simulink model "HIL_Testing_SW_amantest"  (Simulink 7.5)
settings: Solver=ode1  StartTime=0.0  StopTime=Inf  FixedStep=0.001  RelTol=1e-3
PostLoadFcn:
  | , if any(exist('dsrtsu_mdlpostloadfcn', 'file') == [2, 3, 6]), try dsrtsu_mdlpostloadfcn('Execute', bdroot); catch fprintf('Error in PostLoadFcn (dsrtsu_mdlpostloadfcn) for model "%s":\n %s\n', bdroot, lasterr); end, end,
undefined symbols (not defined in the file): CeBSER_Cnt_NumTempAxisPts, ChargeCord, ChargeCord_Control, ChargeToSOCCurr, ChrgCurrLim, CrntSens1Fine, CS_SOCSetPt, CyclerMaxChrgPwr, CyclerMaxDschrgPwr, deltaAhr, Drive_1, Drive_10, Drive_11, Drive_12, Drive_13, Drive_14, Drive_15, Drive_16, Drive_17, Drive_18, Drive_19, Drive_2, Drive_20, Drive_21, Drive_22, Drive_23, Drive_24, Drive_25, Drive_26, Drive_27, Drive_28, Drive_29, Drive_3, Drive_30, Drive_31, Drive_32, Drive_33, Drive_34, Drive_35, Drive_36, Drive_37, Drive_38, Drive_39, Drive_4, Drive_40, Drive_41, Drive_42, Drive_43, Drive_44, Drive_45, Drive_46, Drive_47, Drive_48, Drive_49, Drive_5, Drive_50, Drive_51, Drive_6, Drive_7, Drive_8 ... (+50)
libraries: simulink x129, rtican x50, rti2211sailib x5, rti2211serlib x5, rti2202miolib x3
(part 12 of 23)

== system HIL_Testing_SW_amantest/TX/Tx_Cycler/Send Remote Request B ==
  note: 0x01C3
  Control : Inport  OutDataType=sfix(16)  OutScaling=2^0
  StationID_B1 : Inport  Port=2  OutDataType=sfix(16)  OutScaling=2^0
  StationID_B : Inport  Port=3  OutDataType=sfix(16)  OutScaling=2^0
  Hardware_Version : Inport  Port=4  OutDataType=sfix(16)  OutScaling=2^0
  Enable : EnablePort
  Bus Selector7 : BusSelector  OutputSignals=Channel_Change_B,Control_From_B,Control_To_B
  Change_Control_B : rtican/RTICAN Transmit (TX)   SystemSampleTime=-1  Reserved1=[]  Reserved2=[]  Reserved3=[]  Reserved4=[]  SfcnMessage=[]  Msg_Struct=[]  BoardTypeNo=[]  BoardNo=[]  ChannelNo=[]  Parameters=[]  DialogFcn=[]  UnitName=[]  Revision=[]  UnitValues=[]  DSProperties=struct('RTI',struct('Version',uint32(5),'BlockType',struct('isSLSource',uint8(1),'isSLSink',uint8(1),'isHWSource',uint8(0),'isHWSink',uint8(0),'isSetup',uint8(0),'isInline',uint8(1),'isNonInline',uint8(0),'isInterrupt',uint8(0),'isChannelwise',uint8(0)),'IOBoardType','RTICAN','UnitType','MESSAGE','Identifier','TX','DialogType','MSVC','BlockSet','RTICAN','SlaveProcessor','CAN'))  RTIBlockInterface=struct('InputPortsWidth',int32([1 1 1 1 1 1]),'InputPortsActive',[1 1 1 1 1 1],'InputPortsName',{{'CC_channel_change_B','CC_control_from_B','CC_control_to_B','Station_ID_B','Hardware_ver_ID_B','Station_IDA_B'}},'InputPortsDataType',{{'SS_DOUBLE','SS_DOUBLE','SS_DOUBLE','SS_DOUBLE','SS_DOUBLE','SS_DOUBLE'}},'OutputPortsWidth',int32(1),'OutputPortsActive',1,'OutputPortsName',{{['TX status']}},'DialogFcn','rtican_message_interface_gui','BlockDisplay',{{'','center'}},'IconTransparency','on','InitLevel',3,'BlockName',struct('Token',{{'Change_Control_B'}}),'SampleTime',{{-1}},'TriggerPort',{{'none'}},'EnablePort',{{'none'}})  RTIBlockParameters=struct('BoardTypeNo',{{2211,'OFF',[]}},'BoardNo',{{2,'ON',[1 16]}},'ChannelNo',{{1,'ON',[1 2]}},'Parameters',{{struct('DataFileSupport',struct('DataFileSelectedMaster',1,'DataFileSelectedLocal',1,'DataFileName','c:\data\testing\av900_dbc\av900_mod.dbc|','DataFileDate',{{{['20-Apr-2011 08:23:37']}}},'SelectedFile','av900_dbc\av900_mod.dbc','InterfaceFcn','rtican_dbc_file_parser'),'Options',struct('StatusSelected',1,'TimeSelected',0,'DeltaTimeSelected',0,'DelayTimeSelected',0,'DelayTimeTXCommandSelected',0,'EncodeSetUnusedBitsToOne',0,'EnableMsgLoopback',0,'TriggerPort',struct('Selected',0,'TriggerType',0),'EnablePortSelected',0,'SignalOnPortnameSelected',1,'UserCoding',struct('Selected',0,'InterfaceFile','UserEncodingFile','FcnName','UserEncodeFcn','InportSelected',0,'InportWidth',1,'OutportSelected',0,'OutportWidth',1),'TerminationMsg',struct('Selected',0,'Byte0_7','0'),'InitialMsg',struct('Selected',0,'Byte0_7','0')),'Message',struct('MsgOnBlocknameSelected',1,'MsgName','Change_Control_B','MsgIdFormat',0,'MsgId',451,'MsgLength',8,'NumSignals',6,'SampleTime',-1,'StartTime',struct('Selected',0,'Value',0),'AutoRepeatTime',struct('Selected',0,'Value',0.1),'Timeout',struct('Selected',0,'Value',0.1),'DelayTime',struct('Selected',0,'Value',0.1),'Signal',struct('SgnName',{'CC_channel_change_B','CC_control_from_B','CC_control_to_B','Station_ID_B','Hardware_ver_ID_B','Station_IDA_B'},'SgnStartBit',{0,1,4,8,8,56},'SgnLength',{1,3,3,32,16,8},'SgnType',{0,0,0,0,0,0},'ModeValue',{-1,-1,-1,-1,-1,-1},'DataType',{0,0,0,0,0,0},'ByteLayout',{0,0,0,2,0,0},'Factor',{1,1,1,1,1,1},'Offset',{0,0,0,0,0,0},'SgnComment',{{''},{''},{''},{''},{''},{''}},'SgnUnit',{'code','code','code','code','code','code'},'Min',{0,0,0,0,0,0},'Max',{1,7,7,0,65535,255},'SLDataType',{'SS_DOUBLE','SS_DOUBLE','SS_DOUBLE','SS_DOUBLE','SS_DOUBLE','SS_DOUBLE'}),'MsgIdNumFormat',0,'MsgComment',{{''}}),'Version',1.2,'general',struct('isFromLib',0)),'OFF',[]}},'GroupId',{{struct('Group',{{'RTICAN'}},'No',6,'Behavior',{{'NAMECHANGE'}},'BlockType',{{'SINK'}},'NameChangeFlag',0),'OFF',[]}},'SFcnRTICANMessage',{{struct('MsgType','TX','SFcnPortType','Scalar','MsgName','Change_Control_B','MsgIdFormat','STD','MsgId',451,'MsgLength',8,'NumSignals',6,'SampleTime',-1,'StartTime',struct('Selected','no','Value',0),'AutoRepeatTime',struct('Selected','no','Value',0.1),'Timeout',struct('Selected','no','Value',0.1),'Signal',struct('SgnName',{'CC_channel_change_B','CC_control_from_B','CC_control_to_B','Station_ID_B','Hardware_ver_ID_B','Station_IDA_B'},'SgnStartBit',{0,1,4,8,8,56},'SgnLength',{1,3,3,32,16,8},'SgnType',{'standard','standard','standard','standard','standard','standard'},'ModeValue',{-1,-1,-1,-1,-1,-1},'DataType',{['unsigned int'],['unsigned int'],['unsigned int'],['unsigned int'],['unsigned int'],['unsigned int']},'ByteLayout',{['little endian'],['little endian'],['little endian'],['motorola back.'],['little endian'],['little endian']},'Factor',{1,1,1,1,1,1},'Offset',{0,0,0,0,0,0},'SLDataType',{'SS_DOUBLE','SS_DOUBLE','SS_DOUBLE','SS_DOUBLE','SS_DOUBLE','SS_DOUBLE'}),'StatusSelected','yes','TimeSelected','no','DeltaTimeSelected','no','DelayTimeSelected','no','DelayTimeTXCommandSelected','no','EncodeSetUnusedBitsToOne','no','EnableMsgLoopback','no','TriggerPort',struct('Selected','no','TriggerType',0),'EnablePortSelected','no','UserCoding',struct('Selected','no','InterfaceFile','UserEncodingFile','FcnName','UserEncodeFcn','InportSelected','no','InportWidth',1,'OutportSelected','no','OutportWidth',1),'TerminationMsg',struct('Selected','no','Byte0','0x00','Byte1','0x00','Byte2','0x00','Byte3','0x00','Byte4','0x00','Byte5','0x00','Byte6','0x00','Byte7','0x00'),'InitialMsg',struct('Selected','no','Byte0','0x00','Byte1','0x00','Byte2','0x00','Byte3','0x00','Byte4','0x00','Byte5','0x00','Byte6','0x00','Byte7','0x00'),'BoardType','DS2211','BoardNo',2,'ControllerNo',1),'OFF',[]}},'TLCFileName',{{'rtican_tx_message','OFF',[]}})  RTISFcnParameters=struct('SFcnRTICANMessage','struct','TLCFileName','char')  RTIBlockParaDefault=struct('BoardTypeNo',4302,'BoardNo',1,'ChannelNo',1,'Parameters',struct('DataFileSupport',struct('DataFileSelectedMaster',0,'DataFileSelectedLocal',0,'DataFileName','','DataFileDate','','SelectedFile',['<no file selected>']),'Options',struct('StatusSelected',1,'TimeSelected',1,'DeltaTimeSelected',1,'DelayTimeSelected',1,'DelayTimeTXCommandSelected',0,'EncodeSetUnusedBitsToOne',0,'EnableMsgLoopback',0,'TriggerPort',struct('Selected',0,'TriggerType','rising'),'EnablePortSelected',0,'SignalOnPortnameSelected',1,'UserCoding',struct('Selected',0,'InterfaceFile','UserEncodingFile','FcnName','UserEncodeFcn','InportSelected',0,'InportWidth',1,'OutportSelected',0,'OutportWidth',1),'TerminationMsg',struct('Selected',0,'Byte0_7','0'),'InitialMsg',struct('Selected',0,'Byte0_7','0')),'Message',struct('MsgOnBlocknameSelected',0,'MsgName',['TX Message'],'MsgIdFormat',0,'MsgId',100,'MsgLength',8,'NumSignals',1,'SampleTime',-1,'StartTime',struct('Selected',0,'Value',0),'AutoRepeatTime',struct('Selected',0,'Value',0.1),'Timeout',struct('Selected',0,'Value',0.1),'DelayTime',struct('Selected',0,'Value',0.1),'Signal',struct('SgnName',['TX signal'],'SgnStartBit',0,'SgnLength',8,'SgnType',0,'ModeValue',-1,'DataType',0,'SLDataType','SS_DOUBLE','ByteLayout',0,'Factor',1,'Offset',0,'Min',0,'Max',255,'SgnComment',{{}},'SgnUnit',''),'MsgIdNumFormat',0,'MsgComment',{{''}}),'Version',1.2,'general',struct('isFromLib',1)),'GroupId',struct('Group',{{'RTICAN'}},'No',1,'Behavior',{{'NAMECHANGE'}},'BlockType',{{'SINK'}},'NameChangeFlag',0),'SFcnRTICANMessage',struct('MsgType','TX','MsgName',['TX Message'],'MsgIdFormat','STD','MsgId',100,'MsgLength',2,'NumSignals',1,'SampleTime',-1,'StartTime',struct('Selected','no','Value',0),'AutoRepeatTime',struct('Selected','no','Value',0.1),'Timeout',struct('Selected','no','Value',0.1),'DelayTime',struct('Selected','no','Value',0.1),'Signal',struct('SgnName',['TX signal'],'SgnStartBit',0,'SgnLength',8,'SgnType','standard','ModeValue',-1,'DataType',['unsigned int'],'ByteLayout',['little endian'],'SLDataType','SS_DOUBLE','Factor',1,'Offset',0),'StatusSelected','yes','TimeSelected','yes','DeltaTimeSelected','yes','DelayTimeSelected','yes','EnablePortSelected','no','EnableMsgLoopback','no','DelayTimeTXCommandSelected','no','EncodeSetUnusedBitsToOne','no','UserCoding',struct('Selected','no','InterfaceFile','UserDecodingFile','FcnName','UserDecodeFcn','InportSelected','no','InportWidth',1,'OutportSelected','no','OutportWidth',1),'TerminationMsg',struct('Selected','no','Byte0','0x00','Byte1','0x00','Byte2','0x00','Byte3','0x00','Byte4','0x00','Byte5','0x00','Byte6','0x00','Byte7','0x00'),'InitialMsg',struct('Selected','no','Byte0','0x00','Byte1','0x00','Byte2','0x00','Byte3','0x00','Byte4','0x00','Byte5','0x00','Byte6','0x00','Byte7','0x00'),'TriggerPort',struct('Selected','no','TriggerType','rising'),'BoardType','DS4302','BoardNo',1,'ControllerNo',1,'SFcnPortType','Scalar'),'TLCFileName','rtican_tx_message')
      settings: AttributesFormatString=Group Id: RTICAN6\n
  Constant : Constant  OutDataType=sfix(16)  OutScaling=2^0
  Data Store Write1 : DataStoreWrite  DataStoreName=Remote_Req_B_Sent  SampleTime=-1
  Data Type Conversion{1..5,7} (6 alike) : DataTypeConversion  OutDataType=fixdt(1, 16)  OutScaling=2^0
  Terminator : Terminator
  wires:
  Bus Selector7/1 -> Data Type Conversion7/1  "<Channel_Change_B>"
  Bus Selector7/2 -> Data Type Conversion1/1  "<Control_From_B>"
  Bus Selector7/3 -> Data Type Conversion2/1  "<Control_To_B>"
  StationID_B1/1 -> Data Type Conversion5/1
  Hardware_Version/1 -> Data Type Conversion4/1
  StationID_B/1 -> Data Type Conversion3/1
  Change_Control_B/1 -> Terminator/1
  Control/1 -> Bus Selector7/1
  Constant/1 -> Data Store Write1/1
  Data Type Conversion7/1 -> Change_Control_B/1
  Data Type Conversion1/1 -> Change_Control_B/2
  Data Type Conversion2/1 -> Change_Control_B/3
  Data Type Conversion3/1 -> Change_Control_B/4
  Data Type Conversion4/1 -> Change_Control_B/5
  Data Type Conversion5/1 -> Change_Control_B/6

== system HIL_Testing_SW_amantest/TX/Tx_Cycler/Subsystem ==
  In : Inport
  0x140_Latch_Reset : Constant  Value=0  OutDataType=sfix(16)  OutScaling=2^0
  Comparison4 : RelationalOperator  Operator===  LogicOutDataTypeMode=boolean  OutDataTypeStr=boolean
  Constant Value : Constant  Value=single(1)  OutDataType=sfix(16)  OutScaling=2^0
  Data Type Conversion : DataTypeConversion  OutDataType=sfix(16)  OutScaling=2^0
  Data Type Conversion1 : DataTypeConversion  OutDataType=sfix(16)  OutScaling=2^0
  OurLatchReset : Subsystem
  Out : Outport
  wires:
  OurLatchReset/1(Out1) -> Data Type Conversion/1
  Constant Value/1 -> Comparison4/2
  Comparison4/1 -> OurLatchReset/1(U)
  In/1 -> Comparison4/1
  Data Type Conversion/1 -> Out/1
  Data Type Conversion1/1 -> OurLatchReset/2(Reset)
  0x140_Latch_Reset/1 -> Data Type Conversion1/1

== system HIL_Testing_SW_amantest/TX/Tx_Cycler/TX_ABC_ChA ==
  Control_Value : Inport  OutDataType=sfix(16)  OutScaling=2^0
  Control_Mode : Inport  Port=2  OutDataType=sfix(16)  OutScaling=2^0
  Enable : EnablePort
  Chart : Stateflow chart  TreatAsAtomicUnit=on
  TickTick : Constant  Value=10  OutDataType=sfix(16)  OutScaling=2^0
  msg_0x1A0_Command_A : Subsystem  TreatAsAtomicUnit=on
  msg_0x1A1_Low_Lim_A_out : Subsystem  TreatAsAtomicUnit=on
  msg_0x1A2_Upp_Lim_A_out : Subsystem  TreatAsAtomicUnit=on
  wires:
  Control_Mode/1 -> msg_0x1A0_Command_A/3(Control_Mode)
  Control_Value/1 -> msg_0x1A0_Command_A/2(Control_Value_Proc)
  Chart/3(Trigger_three) -> msg_0x1A2_Upp_Lim_A_out/Enable
  Chart/2(Trigger_two) -> msg_0x1A1_Low_Lim_A_out/Enable
  Chart/1(Trigger_one) -> msg_0x1A0_Command_A/Enable
  Chart/4(Increment) -> [Counter]
  [Counter] -> msg_0x1A2_Upp_Lim_A_out/1(Counter)
  [Counter] -> msg_0x1A1_Low_Lim_A_out/1(Counter)
  [Counter] -> msg_0x1A0_Command_A/1(Counter)
  TickTick/1 -> Chart/1(TickTick)

== system HIL_Testing_SW_amantest/TX/Tx_Cycler/TX_ABC_ChB ==
  Control_Value : Inport  OutDataType=sfix(16)  OutScaling=2^0
  Control_Mode : Inport  Port=2  OutDataType=sfix(16)  OutScaling=2^0
  Enable : EnablePort
  Chart : Stateflow chart  TreatAsAtomicUnit=on
  TickTick : Constant  Value=10  OutDataType=sfix(16)  OutScaling=2^0
  msg_0x1A0_Command_B : Subsystem  TreatAsAtomicUnit=on
  msg_0x1A1_Low_Lim_B_out : Subsystem  TreatAsAtomicUnit=on
  msg_0x1A2_Upp_Lim_B_out : Subsystem  TreatAsAtomicUnit=on
  wires:
  TickTick/1 -> Chart/1(TickTick)
  [Counter] -> msg_0x1A0_Command_B/1(Counter)
  [Counter] -> msg_0x1A1_Low_Lim_B_out/1(Counter)
  [Counter] -> msg_0x1A2_Upp_Lim_B_out/1(Counter)
  Chart/4(Increment) -> [Counter]
  Chart/1(Trigger_one) -> msg_0x1A0_Command_B/Enable
  Chart/2(Trigger_two) -> msg_0x1A1_Low_Lim_B_out/Enable
  Chart/3(Trigger_three) -> msg_0x1A2_Upp_Lim_B_out/Enable
  Control_Value/1 -> msg_0x1A0_Command_B/2(Control_Value_Proc)
  Control_Mode/1 -> msg_0x1A0_Command_B/3(Control_Mode)

== system HIL_Testing_SW_amantest/HWO/TX HVEM/ChargeCord_Control/110 ==
  Action Port : ActionPort  ActionType=then
  Constant : Constant  OutDataTypeMode=uint32  OutDataType=sfix(16)  OutScaling=2^0  OutDataTypeStr=uint32
  Out1 : Outport  OutDataType=sfix(16)  OutScaling=2^0  InitialOutput=1
  wires:
  Constant/1 -> Out1/1

== system HIL_Testing_SW_amantest/HWO/TX HVEM/ChargeCord_Control/220 ==
  Action Port : ActionPort  ActionType=elseif
  Constant : Constant  Value=2  OutDataTypeMode=uint32  OutDataType=sfix(16)  OutScaling=2^0  OutDataTypeStr=uint32
  Out1 : Outport  OutDataType=sfix(16)  OutScaling=2^0  InitialOutput=2
  wires:
  Constant/1 -> Out1/1

== system HIL_Testing_SW_amantest/HWO/TX HVEM/ChargeCord_Control/Cord Connected ==
  Proximity : Inport  OutDataType=sfix(16)  OutScaling=2^0
  Freq1 : Inport  Port=2  OutDataType=sfix(16)  OutScaling=2^0
  AC_Enable : Inport  Port=3  OutDataType=sfix(16)  OutScaling=2^0
  Outlet Type : Inport  Port=4  OutDataType=sfix(16)  OutScaling=2^0
  PrcsdVolt_Freq1 : Inport  Port=5  OutDataType=sfix(16)  OutScaling=2^0
  Action Port : ActionPort  ActionType=then
  110 Connected : Subsystem  TreatAsAtomicUnit=on
  110_Current : Constant  Value=11  OutDataType=sfix(16)  OutScaling=2^0  OutDataTypeStr=Inherit: Inherit via back propagation
  110_DC : Constant  Value=20  OutDataType=sfix(16)  OutScaling=2^0  OutDataTypeStr=Inherit: Inherit via back propagation
  110_Temp : Constant  Value=22  OutDataType=sfix(16)  OutScaling=2^0  OutDataTypeStr=Inherit: Inherit via back propagation
  110_Volts : Constant  Value=110  OutDataType=sfix(16)  OutScaling=2^0  OutDataTypeStr=Inherit: Inherit via back propagation
  220 Connected : Subsystem  TreatAsAtomicUnit=on
  220_Current : Constant  Value=15  OutDataType=sfix(16)  OutScaling=2^0  OutDataTypeStr=Inherit: Inherit via back propagation
  220_DC : Constant  Value=22  OutDataType=sfix(16)  OutScaling=2^0  OutDataTypeStr=Inherit: Inherit via back propagation
  220_Temp : Constant  Value=22  OutDataType=sfix(16)  OutScaling=2^0  OutDataTypeStr=Inherit: Inherit via back propagation
  220_Volts : Constant  Value=220  OutDataType=sfix(16)  OutScaling=2^0  OutDataTypeStr=Inherit: Inherit via back propagation
  AC Enabled : Subsystem  TreatAsAtomicUnit=on
  AC Not Enabled : Subsystem  TreatAsAtomicUnit=on
  ACNotEnableD_Current : Constant  Value=0  OutDataType=sfix(16)  OutScaling=2^0  OutDataTypeStr=Inherit: Inherit via back propagation
  ACNotEnabled_Volts : Constant  Value=0  OutDataType=sfix(16)  OutScaling=2^0  OutDataTypeStr=Inherit: Inherit via back propagation
  If1 : If  IfExpression=u1==1  ElseIfExpressions=u1==2  ZeroCross=off
  If2 : If  IfExpression=u1==1  ZeroCross=off
  Merge{,1..3,6} (5 alike) : Merge  Inputs=3
  Merge4 : Merge
  Merge5 : Merge
  Not Connected : Subsystem  TreatAsAtomicUnit=on
  NotConnecteD_Temp : Constant  Value=-40  OutDataType=sfix(16)  OutScaling=2^0  OutDataTypeStr=Inherit: Inherit via back propagation
  NotConnected_Current : Constant  Value=0  OutDataType=sfix(16)  OutScaling=2^0  OutDataTypeStr=Inherit: Inherit via back propagation
  NotConnected_DC : Constant  Value=10  OutDataType=sfix(16)  OutScaling=2^0  OutDataTypeStr=Inherit: Inherit via back propagation
  NotConnected_Volts : Constant  Value=0  OutDataType=sfix(16)  OutScaling=2^0  OutDataTypeStr=Inherit: Inherit via back propagation
  ChargeCrdPresent : Outport  OutDataType=sfix(16)  OutScaling=2^0
  DC : Outport  Port=2  OutDataType=sfix(16)  OutScaling=2^0
  Freq : Outport  Port=3  OutDataType=sfix(16)  OutScaling=2^0
  Voltage : Outport  Port=4  OutDataType=sfix(16)  OutScaling=2^0  InitialOutput=0
  Current : Outport  Port=5  OutDataType=sfix(16)  OutScaling=2^0  InitialOutput=0
  Temp : Outport  Port=6  OutDataType=sfix(16)  OutScaling=2^0
  PrcsdVolt_DC : Outport  Port=7  OutDataType=sfix(16)  OutScaling=2^0
  PrcsdVolt_Freq : Outport  Port=8  OutDataType=sfix(16)  OutScaling=2^0
  wires:
  If2/1 -> AC Enabled/Action
  AC Not Enabled/2(Current_out) -> Merge5/2
  AC Not Enabled/1(Volt_out) -> Merge4/2
  ACNotEnableD_Current/1 -> AC Not Enabled/2(Current_in)
  ACNotEnabled_Volts/1 -> AC Not Enabled/1(Volt_in)
  If1/1 -> 110 Connected/Action
  [Current] -> AC Enabled/2(Current_in)
  [Voltage] -> AC Enabled/1(Volt_in)
  Merge1/1 -> [Current]
  Merge/1 -> [Voltage]
  AC Enabled/2(Current_out) -> Merge5/1
  AC Enabled/1(Volt_out) -> Merge4/1
  Merge5/1 -> Current/1
  Merge4/1 -> Voltage/1
  Merge3/1 -> DC/1
  Merge2/1 -> Temp/1
  If2/2 -> AC Not Enabled/Action
  AC_Enable/1 -> If2/1
  Proximity/1 -> ChargeCrdPresent/1
  Freq1/1 -> Freq/1
  Outlet Type/1 -> If1/1
  110_Volts/1 -> 110 Connected/1(Volt_in)
  If1/2 -> 220 Connected/Action
  If1/3 -> Not Connected/Action
  110_Current/1 -> 110 Connected/2(Current_in)
  110_Temp/1 -> 110 Connected/3(Temp_in)
  220_Volts/1 -> 220 Connected/1(Volt_in)
  220_Current/1 -> 220 Connected/2(Current_in)
  220_Temp/1 -> 220 Connected/3(Temp_in)
  NotConnected_Volts/1 -> Not Connected/1(Volt_in)
  NotConnected_Current/1 -> Not Connected/2(Current_in)
  NotConnecteD_Temp/1 -> Not Connected/3(Temp_in)
  110 Connected/1(Volt_out) -> Merge/1
  110 Connected/2(Current_out) -> Merge1/1
  220 Connected/1(Volt_out) -> Merge/2
  220 Connected/2(Current_out) -> Merge1/2
  110 Connected/3(Temp_out) -> Merge2/1
  220 Connected/3(Temp_out) -> Merge2/2
  Not Connected/1(Volt_out) -> Merge/3
  Not Connected/2(Current_out) -> Merge1/3
  Not Connected/3(Temp_out) -> Merge2/3
  220_DC/1 -> 220 Connected/4(DC_in)
  110 Connected/4(DC_Out) -> Merge3/1
  110_DC/1 -> 110 Connected/4(DC_in)
  220 Connected/4(DC_Out) -> Merge3/2
  NotConnected_DC/1 -> Not Connected/4(DC_in)
  Not Connected/4(DC_Out) -> Merge3/3
  Merge6/1 -> PrcsdVolt_DC/1
  110 Connected/5(PrcsdVolt_DC) -> Merge6/1
  220 Connected/5(PrcsdVolt_DC) -> Merge6/2
  Not Connected/5(PrcsdVolt_DC) -> Merge6/3
  PrcsdVolt_Freq1/1 -> PrcsdVolt_Freq/1

== system HIL_Testing_SW_amantest/HWO/TX HVEM/ChargeCord_Control/Cord Not Connected ==
  Proximity : Inport  OutDataType=sfix(16)  OutScaling=2^0
  DC_in : Inport  Port=2  OutDataType=sfix(16)  OutScaling=2^0
  Freq_in : Inport  Port=3  OutDataType=sfix(16)  OutScaling=2^0
  Voltage_in : Inport  Port=4  OutDataType=sfix(16)  OutScaling=2^0
  Current_in : Inport  Port=5  OutDataType=sfix(16)  OutScaling=2^0
  Temp_in : Inport  Port=6  OutDataType=sfix(16)  OutScaling=2^0
  PrcsdVolt_DC_in : Inport  Port=7  OutDataType=sfix(16)  OutScaling=2^0
  PrcsdVolt_Freq_in : Inport  Port=8  OutDataType=sfix(16)  OutScaling=2^0
  Action Port : ActionPort  ActionType=else
  ChargeCrdPresent : Outport  OutDataType=sfix(16)  OutScaling=2^0
  DC_out : Outport  Port=2  OutDataType=sfix(16)  OutScaling=2^0
  Freq : Outport  Port=3  OutDataType=sfix(16)  OutScaling=2^0
  Voltage : Outport  Port=4  OutDataType=sfix(16)  OutScaling=2^0
  Current : Outport  Port=5  OutDataType=sfix(16)  OutScaling=2^0
  Temp : Outport  Port=6  OutDataType=sfix(16)  OutScaling=2^0
  PrcsdVolt_DC : Outport  Port=7  OutDataType=sfix(16)  OutScaling=2^0
  PrcsdVolt_Freq : Outport  Port=8  OutDataType=sfix(16)  OutScaling=2^0
  wires:
  Temp_in/1 -> Temp/1
  Current_in/1 -> Current/1
  Freq_in/1 -> Freq/1
  Voltage_in/1 -> Voltage/1
  Proximity/1 -> ChargeCrdPresent/1
  DC_in/1 -> DC_out/1
  PrcsdVolt_DC_in/1 -> PrcsdVolt_DC/1
  PrcsdVolt_Freq_in/1 -> PrcsdVolt_Freq/1

== system HIL_Testing_SW_amantest/HWO/TX HVEM/ChargeCord_Control/Disconnected ==
  Action Port : ActionPort  ActionType=else
  Constant : Constant  Value=0  OutDataTypeMode=uint32  OutDataType=sfix(16)  OutScaling=2^0  OutDataTypeStr=uint32
  Out1 : Outport  OutDataType=sfix(16)  OutScaling=2^0  InitialOutput=3
  wires:
  Constant/1 -> Out1/1

== system HIL_Testing_SW_amantest/HWO/TX HVEM/ChargeCord_Control/OurLatchReset ==
  U : Inport  OutDataType=fixdt(1, 16)  OutScaling=2^0
  Reset : Inport  Port=2  OutDataType=fixdt(1, 16)  OutScaling=2^0
  Logical Operator : Logic  Operator=NOT  AllPortsSameDT=off  OutDataTypeMode=boolean  LogicDataType=fixdt(0, 8)  OutDataTypeStr=boolean
  Logical Operator1 : Logic  Operator=OR  AllPortsSameDT=off  OutDataTypeMode=boolean  LogicDataType=fixdt(0, 8)  OutDataTypeStr=boolean
  Logical Operator2 : Logic  AllPortsSameDT=off  OutDataTypeMode=boolean  LogicDataType=fixdt(0, 8)  OutDataTypeStr=boolean
  Unit Delay : UnitDelay  SampleTime=-1
  Out1 : Outport  OutDataType=fixdt(1, 16)  OutScaling=2^0
  wires:
  Unit Delay/1 -> Logical Operator2/2
  Logical Operator1/1 -> Unit Delay/1, Out1/1
  U/1 -> Logical Operator1/1
  Logical Operator2/1 -> Logical Operator1/2
  Logical Operator/1 -> Logical Operator2/1
  Reset/1 -> Logical Operator/1

== system HIL_Testing_SW_amantest/HWO/TX HVEM/ChargeCord_Control/OurLatchReset1 ==
  U : Inport  OutDataType=fixdt(1, 16)  OutScaling=2^0
  Reset : Inport  Port=2  OutDataType=fixdt(1, 16)  OutScaling=2^0
  Logical Operator : Logic  Operator=NOT  AllPortsSameDT=off  OutDataTypeMode=boolean  LogicDataType=fixdt(0, 8)  OutDataTypeStr=boolean
  Logical Operator1 : Logic  Operator=OR  AllPortsSameDT=off  OutDataTypeMode=boolean  LogicDataType=fixdt(0, 8)  OutDataTypeStr=boolean
  Logical Operator2 : Logic  AllPortsSameDT=off  OutDataTypeMode=boolean  LogicDataType=fixdt(0, 8)  OutDataTypeStr=boolean
  Unit Delay : UnitDelay  SampleTime=-1
  Out1 : Outport  OutDataType=fixdt(1, 16)  OutScaling=2^0
  wires:
  Reset/1 -> Logical Operator/1
  Logical Operator/1 -> Logical Operator2/1
  Logical Operator2/1 -> Logical Operator1/2
  U/1 -> Logical Operator1/1
  Logical Operator1/1 -> Out1/1, Unit Delay/1
  Unit Delay/1 -> Logical Operator2/2

== system HIL_Testing_SW_amantest/LionsHeart/FeaturePresentation/Ahr_Integration/Clear Ahr ==
  note: Clear Ahr
  Enable : EnablePort
  Constant Value{,1..3} (4 alike) : Constant  Value=0  OutDataType=sfix(16)  OutScaling=2^0
  Data Store Write : DataStoreWrite  DataStoreName=Ahr  SampleTime=-1
  Data Store Write1 : DataStoreWrite  DataStoreName=Whr  SampleTime=-1
  Data Store Write2 : DataStoreWrite  DataStoreName=Whr_PackSens  SampleTime=-1
  Data Store Write3 : DataStoreWrite  DataStoreName=Ahr_PackSens  SampleTime=-1
  wires:
  Constant Value/1 -> Data Store Write/1
  Constant Value1/1 -> Data Store Write1/1
  Constant Value2/1 -> Data Store Write2/1
  Constant Value3/1 -> Data Store Write3/1

== system HIL_Testing_SW_amantest/LionsHeart/FeaturePresentation/Ahr_Integration/Cycler_Ahr ==
  Current : Inport  OutDataType=sfix(16)  OutScaling=2^0
  Voltage : Inport  Port=2  OutDataType=sfix(16)  OutScaling=2^0
  Constant Value : Constant  Value=0.001  OutDataType=sfix(16)  OutScaling=2^0
  Constant Value1 : Constant  Value=3600  OutDataType=sfix(16)  OutScaling=2^0
  Data Store Read1 : DataStoreRead  DataStoreName=SOC  SampleTime=0
  Data Store Read2 : DataStoreRead  DataStoreName=PackCapacity  SampleTime=0
  Data Store Read3 : DataStoreRead  DataStoreName=Ahr  SampleTime=0
  Data Store Read4 : DataStoreRead  DataStoreName=Whr  SampleTime=0
  Divide : Constant  Value=2  OutDataType=sfix(16)  OutScaling=2^0
  Product : Product  OutDataType=sfix(16)  OutScaling=2^0  RndMeth=Zero
  Product1 : Product  Inputs=*/  OutDataType=sfix(16)  OutScaling=2^0  RndMeth=Zero
  Product2 : Product  Inputs=*/  OutDataType=sfix(16)  OutScaling=2^0  RndMeth=Zero
  Product3 : Product  Inputs=*/  OutDataType=sfix(16)  OutScaling=2^0  RndMeth=Zero
  Product4 : Product  OutDataType=sfix(16)  OutScaling=2^0  RndMeth=Zero
  Sum{,1..3} (4 alike) : Sum  OutDataType=sfix(16)  OutScaling=2^0  RndMeth=Zero
  Unit Delay : UnitDelay  SampleTime=-1
  SOC : Outport  OutDataType=fixdt(1, 16)  OutScaling=2^0
  Ahr : Outport  Port=2  OutDataType=fixdt(1, 16)  OutScaling=2^0
  Whr : Outport  Port=3  OutDataType=fixdt(1, 16)  OutScaling=2^0
  wires:
  [Inst_SOC] -> Sum2/1
  Product2/1 -> Product/1
  Constant Value/1 -> Product/2
  Product/1 -> Product1/1
  Constant Value1/1 -> Product1/2
  Divide/1 -> Product2/2
  Sum1/1 -> Product2/1
  Current/1 -> Sum1/1, Unit Delay/1
  Unit Delay/1 -> Sum1/2
  Product1/1 -> Sum/1, Product3/1, Product4/1
  Product3/1 -> [Inst_SOC]
  Data Store Read2/1 -> Product3/2
  Sum/1 -> Ahr/1
  Voltage/1 -> Product4/2
  Product4/1 -> Sum3/1
  Sum3/1 -> Whr/1
  Data Store Read1/1 -> Sum2/2
  Sum2/1 -> SOC/1
  Data Store Read3/1 -> Sum/2
  Data Store Read4/1 -> Sum3/2

== system HIL_Testing_SW_amantest/LionsHeart/FeaturePresentation/Ahr_Integration/Lookup_SOC ==
  note: SOC Reset
  Voltage : Inport  OutDataType=sfix(16)  OutScaling=2^0
  BatTemp : Inport  Port=2  OutDataType=sfix(16)  OutScaling=2^0
  PackVoltage : Inport  Port=3  OutDataType=sfix(16)  OutScaling=2^0
  Enable : EnablePort
  Data Store Read1 : DataStoreRead  DataStoreName=NumberOfCells  SampleTime=-1
  Data Store Read2 : DataStoreRead  DataStoreName=NumberOfCells  SampleTime=-1
  Data Store Write1 : DataStoreWrite  DataStoreName=SOC  SampleTime=-1
  Data Store Write2 : DataStoreWrite  DataStoreName=SOC_PackSens  SampleTime=-1
  Data Type Conversion{1..2,5..6} (4 alike) : DataTypeConversion  OutDataTypeMode=single  OutDataType=sfix(16)  OutScaling=2^0  OutDataTypeStr=single
  Data Type Conversion3 : DataTypeConversion  OutDataTypeMode=double  OutDataType=sfix(16)  OutScaling=2^0  OutDataTypeStr=double
  Data Type Conversion4 : DataTypeConversion  OutDataTypeMode=double  OutDataType=sfix(16)  OutScaling=2^0  OutDataTypeStr=double
  Divide1 : Product  Inputs=*/  OutDataType=sfix(16)  OutScaling=2^-10
  Divide2 : Product  Inputs=*/  OutDataType=sfix(16)  OutScaling=2^-10
  OCV_Table : Lookup2D  RowIndex=KnBSER_T_SOCv_Row  ColumnIndex=KnBSER_U_SOCv_Col  Table=KtBSER_Pct_SOCv  OutDataType=sfix(16)  OutScaling=2^0
  OCV_TablePack : Lookup2D  RowIndex=KnBSER_T_SOCv_Row  ColumnIndex=KnBSER_U_SOCv_Col  Table=KtBSER_Pct_SOCv  OutDataType=sfix(16)  OutScaling=2^0
  wires:
  Voltage/1 -> Divide1/1
  Data Store Read1/1 -> Divide1/2
  Divide1/1 -> Data Type Conversion2/1
  OCV_Table/1 -> Data Type Conversion3/1
  Data Type Conversion1/1 -> OCV_Table/1
  Data Type Conversion2/1 -> OCV_Table/2
  Data Type Conversion3/1 -> Data Store Write1/1
  BatTemp/1 -> [BatTemp]
  OCV_TablePack/1 -> Data Type Conversion4/1
  Data Type Conversion4/1 -> Data Store Write2/1
  Divide2/1 -> Data Type Conversion6/1
  PackVoltage/1 -> Divide2/1
  Data Store Read2/1 -> Divide2/2
  [BatTemp] -> Data Type Conversion5/1
  [BatTemp] -> Data Type Conversion1/1
  Data Type Conversion5/1 -> OCV_TablePack/1
  Data Type Conversion6/1 -> OCV_TablePack/2

== system HIL_Testing_SW_amantest/LionsHeart/FeaturePresentation/Ahr_Integration/Pack_Ahr ==
  PackCurrent : Inport  OutDataType=sfix(16)  OutScaling=2^0
  PackVoltage : Inport  Port=2  OutDataType=sfix(16)  OutScaling=2^0
  Constant Value : Constant  Value=0.001  OutDataType=sfix(16)  OutScaling=2^0
  Constant Value1 : Constant  Value=3600  OutDataType=sfix(16)  OutScaling=2^0
  Data Store Read1 : DataStoreRead  DataStoreName=SOC_PackSens  SampleTime=0
  Data Store Read2 : DataStoreRead  DataStoreName=PackCapacity  SampleTime=0
  Data Store Write : DataStoreWrite  DataStoreName=SOC_PackSens  SampleTime=-1
  Data Store Write1 : DataStoreWrite  DataStoreName=Ahr_PackSens  SampleTime=-1
  Data Store Write2 : DataStoreWrite  DataStoreName=Whr_PackSens  SampleTime=-1
  Divide : Constant  Value=2  OutDataType=sfix(16)  OutScaling=2^0
  Product : Product  OutDataType=sfix(16)  OutScaling=2^0  RndMeth=Zero
  Product1 : Product  Inputs=*/  OutDataType=sfix(16)  OutScaling=2^0  RndMeth=Zero
  Product2 : Product  Inputs=*/  OutDataType=sfix(16)  OutScaling=2^0  RndMeth=Zero
  Product3 : Product  Inputs=*/  OutDataType=sfix(16)  OutScaling=2^0  RndMeth=Zero
  Product4 : Product  OutDataType=sfix(16)  OutScaling=2^0  RndMeth=Zero
  Sum{,1..3} (4 alike) : Sum  OutDataType=sfix(16)  OutScaling=2^0  RndMeth=Zero
  Unit Delay : UnitDelay  SampleTime=-1
  Unit Delay2 : UnitDelay  SampleTime=-1
  Unit Delay3 : UnitDelay  SampleTime=-1
  wires:
  Sum2/1 -> Data Store Write/1
  [Inst_SOC] -> Sum2/1
  Product2/1 -> Product/1
  Constant Value/1 -> Product/2
  Product/1 -> Product1/1
  Constant Value1/1 -> Product1/2
  Divide/1 -> Product2/2
  Sum1/1 -> Product2/1
  PackCurrent/1 -> Sum1/1, Unit Delay/1
  Unit Delay/1 -> Sum1/2
  Product1/1 -> Sum/1, Product3/1, Product4/1
  Product3/1 -> [Inst_SOC]
  Data Store Read2/1 -> Product3/2
  Sum/1 -> Data Store Write1/1, Unit Delay2/1
  Unit Delay2/1 -> Sum/2
  PackVoltage/1 -> Product4/2
  Product4/1 -> Sum3/1
  Unit Delay3/1 -> Sum3/2
  Sum3/1 -> Data Store Write2/1, Unit Delay3/1
  Data Store Read1/1 -> Sum2/2

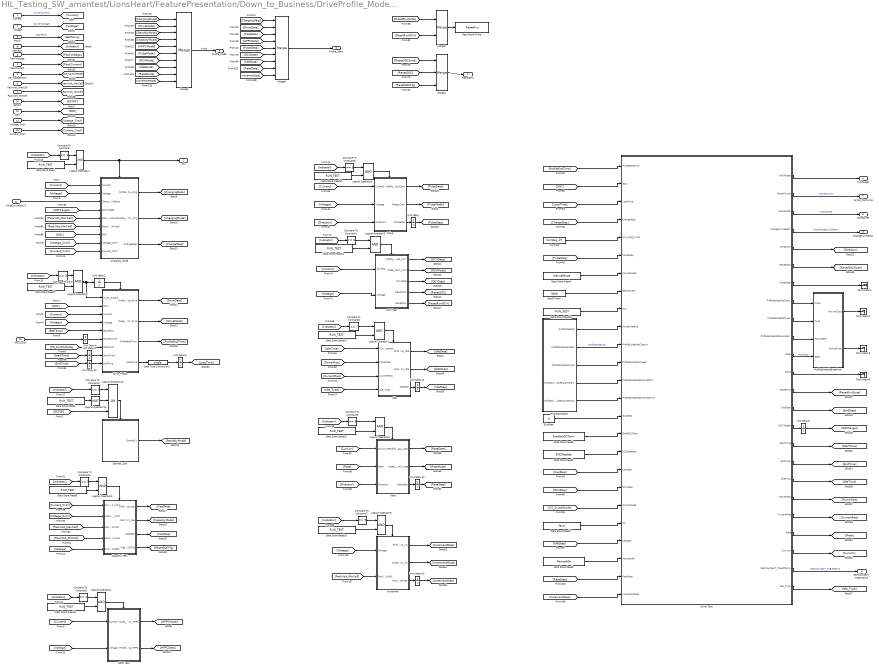
== system HIL_Testing_SW_amantest/LionsHeart/FeaturePresentation/Down_to_Business/DriveProfile_ModeControl ==
  Current : Inport  OutDataType=sfix(16)  OutScaling=2^0
  Voltage : Inport  Port=2  OutDataType=sfix(16)  OutScaling=2^0
  Temp : Inport  Port=3  OutDataType=sfix(16)  OutScaling=2^0
  PackVoltage : Inport  Port=4  OutDataType=sfix(16)  OutScaling=2^0
  PackCurrent : Inport  Port=5  OutDataType=sfix(16)  OutScaling=2^0
  PackVolt_MaxCell : Inport  Port=6  OutDataType=sfix(16)  OutScaling=2^0
  PackVolt_MinCell : Inport  Port=7  OutDataType=sfix(16)  OutScaling=2^0
  Indicator : Inport  Port=8  OutDataType=sfix(16)  OutScaling=2^0
  CS_ModeSwitch : Inport  Port=9  OutDataType=sfix(16)  OutScaling=2^0
  ESTOP : Inport  Port=10  OutDataType=sfix(16)  OutScaling=2^0
  ChrgCurrSelect_F : Inport  Port=11  OutDataType=sfix(16)  OutScaling=2^0
  SOC : Inport  Port=12  OutDataType=sfix(16)  OutScaling=2^0
  PwrCycle : Inport  Port=13  OutDataType=sfix(16)  OutScaling=2^0
  Voltage_Cntrl : Inport  Port=14  OutDataType=sfix(16)  OutScaling=2^0
  Current_Cntrl : Inport  Port=15  OutDataType=sfix(16)  OutScaling=2^0
  Capacity Test : Subsystem
  Charging_Mode : Subsystem
  Compare To Constant : simulink/Logic and Bit Operations/Compare To Constant  SystemSampleTime=-1  relop===  const=1  LogicOutDataTypeMode=boolean
  Compare To Constant1 : simulink/Logic and Bit Operations/Compare To Constant  SystemSampleTime=-1  relop===  const=4  LogicOutDataTypeMode=boolean
  Compare To Constant2 : simulink/Logic and Bit Operations/Compare To Constant  SystemSampleTime=-1  relop===  const=2  LogicOutDataTypeMode=uint8
  Compare To Constant3 : simulink/Logic and Bit Operations/Compare To Constant  SystemSampleTime=-1  relop===  const=3  LogicOutDataTypeMode=boolean
  Compare To Constant4 : simulink/Logic and Bit Operations/Compare To Constant  SystemSampleTime=-1  relop===  const=6  LogicOutDataTypeMode=boolean
  Compare To Constant5 : simulink/Logic and Bit Operations/Compare To Constant  SystemSampleTime=-1  relop===  const=5  LogicOutDataTypeMode=boolean
  Compare To Constant6 : simulink/Logic and Bit Operations/Compare To Constant  SystemSampleTime=-1  relop===  const=7  LogicOutDataTypeMode=boolean
  Compare To Constant7 : simulink/Logic and Bit Operations/Compare To Constant  SystemSampleTime=-1  relop===  const=9  LogicOutDataTypeMode=boolean
  Compare To Constant9 : simulink/Logic and Bit Operations/Compare To Constant  SystemSampleTime=-1  relop===  const=8  LogicOutDataTypeMode=boolean
  Compare To Zero : simulink/Logic and Bit Operations/Compare To Zero  SystemSampleTime=-1  relop===  LogicOutDataTypeMode=boolean
  Data Store Read{,1,7..8,11..16,18} (11 alike) : DataStoreRead  DataStoreName=RUN_TEST  SampleTime=0
  Data Store Read17 : DataStoreRead  DataStoreName=fault  SampleTime=0
  Data Store Read4 : DataStoreRead  DataStoreName=ManualMode  SampleTime=0
  Data Store Read5 : DataStoreRead  DataStoreName=SOCDeplete  SampleTime=0
  Data Store Read6 : DataStoreRead  DataStoreName=EnableSOCTerm  SampleTime=0
  Data Store Read9 : DataStoreRead  DataStoreName=ManualIdle  SampleTime=0
  Data Store Write : DataStoreWrite  DataStoreName=ResetRun  SampleTime=-1
  Data Type Conversion1 : DataTypeConversion  OutDataTypeMode=single  OutDataType=fixdt(1, 16)  OutScaling=2^0  OutDataTypeStr=single
  Drive_Profile : Subsystem
  HPPC Test : Subsystem
  Idle : Subsystem
  Increment : Subsystem
  Logical Operator{1..9} (9 alike) : Logic  AllPortsSameDT=off  OutDataTypeMode=boolean  LogicDataType=fixdt(0, 8)  OutDataTypeStr=boolean
  Logical Operator10 : Logic  Operator=OR  Inputs=3  AllPortsSameDT=off  OutDataTypeMode=boolean  LogicDataType=fixdt(0, 8)  OutDataTypeStr=boolean
  Logical Operator11 : Logic  Operator=NOT  AllPortsSameDT=off  OutDataTypeMode=boolean  LogicDataType=fixdt(0, 8)  OutDataTypeStr=boolean
  Merge1 : Merge  Inputs=10
  Merge2 : Merge  Inputs=3
  Merge3 : Merge
  Merge4 : Merge  Inputs=9
  OCV Test : Subsystem
  ProfileSchedule : Subsystem
  ProfileScheduleBreakout : Subsystem
  Pulse : Subsystem
  Rate : Subsystem
  RestTimeIn : Constant  Tag=R12-1  Value=3600  OutDataTypeMode=double  OutDataType=sfix(16)  OutScaling=2^0  OutDataTypeStr=double
  Scirpt Test : Stateflow chart  TreatAsAtomicUnit=on
  SkipStep : Constant  Value=0  VectorParams1D=off  OutDataTypeMode=boolean  OutDataType=Enum: ProfileScheduling  ConRadixGroup=Best Precision: Vector-wise  OutDataTypeStr=boolean
  Standby_Sub : Subsystem  TreatAsAtomicUnit=on
  Terminator{1,3..4,6} (4 alike) : Terminator
  Unit Delay{,2,4..5,9..11,13..14} (9 alike) : UnitDelay  SampleTime=-1
  Unit Delay8 : UnitDelay  X0=1  SampleTime=-1
  simstep : Constant  Tag=R12-1  Value=SimStep_dT  OutDataTypeMode=double  OutDataType=sfix(16)  OutScaling=2^0  OutDataTypeStr=double
  Profile_Data : Outport  OutDataType=sfix(16)  OutScaling=2^0
  CM : Outport  Port=2  OutDataType=sfix(16)  OutScaling=2^0
  ResetSOC : Outport  Port=3  OutDataType=fixdt(1, 16)  OutScaling=2^0
  VoltTarget : Outport  Port=4  OutDataType=fixdt(1, 16)  OutScaling=2^0
  IndicatorSF : Outport  Port=5  OutDataType=fixdt(1, 16)  OutScaling=2^0
  Profile_Mode : Outport  Port=6  OutDataType=sfix(16)  OutScaling=2^0
  Script_PwrCycle : Outport  Port=7  OutDataType=fixdt(1, 16)  OutScaling=2^0
  ChargeCurrSelect : Outport  Port=8  OutDataType=fixdt(1, 16)  OutScaling=2^0
  SetChamberT_ToBatTemp : Outport  Port=9  OutDataType=fixdt(1, 16)  OutScaling=2^0
  wires:
  Merge4/1 -> Profile_Data/1
  Current/1 -> [Current]  "CyclerCurrent"
  Voltage/1 -> [Voltage]  "CyclerVoltage"
  Temp/1 -> [BatTemp]  "BatTemp"
  [Current] -> Charging_Mode/1(Current)
  [Voltage] -> Charging_Mode/2(Voltage)
  [Current] -> Drive_Profile/3(Current)
  [Voltage] -> Drive_Profile/4(Voltage)
  [BatTemp] -> Drive_Profile/5(BatTemp)
  [SOC] -> Drive_Profile/2(SOC)
  [Indicator] -> Compare To Constant/1
  [Indicator] -> Compare To Zero/1
  [Indicator] -> Compare To Constant2/1
  Charging_Mode/1(Profile_Data_chrg) -> [ChargingData]
  Charging_Mode/2(Mode_Cntrl_chrg) -> [ChargingMode]
  Standby_Sub/1(Standby1) -> [StandbyMode]
  [Current_Cntrl] -> Capacity Test/1(Current_Cntrl)
  [Voltage_Cntrl] -> Capacity Test/2(Voltage_Cntrl)
  [Indicator] -> Compare To Constant3/1
  Capacity Test/1(Profile_Data_cap) -> [CapData]
  Capacity Test/2(Mode_Cntrl_cap) -> [CapacityMode]
  Compare To Constant/1 -> Logical Operator1/1
  Logical Operator1/1 -> Charging_Mode/Enable, CM/1
  Data Store Read/1 -> Logical Operator1/2
  Compare To Zero/1 -> Logical Operator2/1
  Logical Operator2/1 -> Drive_Profile/1(cycle_enable), Unit Delay2/1
  Compare To Constant3/1 -> Logical Operator3/1
  Drive_Profile/1(Profile_Data_drive) -> [DriveData]
  Drive_Profile/2(Mode_Cntrl_drive) -> [DriveMode]
  Logical Operator3/1 -> Capacity Test/Enable
  [Current] -> HPPC Test/1(Current)
  [Voltage] -> HPPC Test/2(Voltage)
  [Indicator] -> Compare To Constant1/1
  Compare To Constant1/1 -> Logical Operator4/1
  Logical Operator4/1 -> HPPC Test/Enable
  HPPC Test/1(Mode_Cntrl_HPPC) -> [HPPCMode]
  HPPC Test/2(Profile_Data_HPPC) -> [HPPCData]
  ChrgCurrSelect_F/1 -> Charging_Mode/3(ChargeCurrSelect)
  [ProfileEndTime] -> Scirpt Test/1(ProfileEndTime)
  Scirpt Test/2(PowerCycle) -> Script_PwrCycle/1  "PowerCycle"
  PwrCycle/1 -> Unit Delay4/1
  Scirpt Test/4(ChargeCurrSelect) -> ChargeCurrSelect/1  "OutChargeCurrSelect"
  Charging_Mode/3(ChargeStep) -> [ChargeStep]
  simstep/1 -> Scirpt Test/5(sim_step_time)
  [Current] -> Pulse/1(Current)
  [Voltage] -> Pulse/2(Voltage)
  [Indicator] -> Compare To Constant5/1
  Pulse/1(Profile_Data_Pulse) -> [PulseData]
  Pulse/2(Mode_Cntrl) -> [PulseMode]
  Compare To Constant5/1 -> Logical Operator5/1
  Logical Operator5/1 -> Pulse/Enable
  Scirpt Test/5(Direction) -> [Direction]
  [Direction] -> Pulse/3(Direction)
  Pulse/3(PulseStep) -> Unit Delay/1
  Unit Delay2/1 -> Drive_Profile/Enable
  Unit Delay/1 -> [PulseStep]
  Unit Delay4/1 -> Drive_Profile/6(PowerCycle)
  Drive_Profile/3(ProfileEndTime) -> [ProfileEndTime]
  RestTimeIn/1 -> Scirpt Test/8(RestTimeIn)
  Data Store Read18/1 -> Scirpt Test/9(Run)
  Data Type Conversion1/1 -> Unit Delay8/1
  Unit Delay8/1 -> [LoopTime]
  Drive_Profile/4(LoopTime) -> Data Type Conversion1/1
  [LoopTime] -> Scirpt Test/3(LoopTime)
  PackVoltage/1 -> [PackVoltage]
  PackCurrent/1 -> [PackCurrent]
  Data Store Read4/1 -> Scirpt Test/7(ManualMode)
  ProfileSchedule/2(ProfileScheduleClass) -> Scirpt Test/11(ProfileScheduleClassIn)  "ProfileSchedule"
  [ChargeStep] -> Scirpt Test/4(ChargeStep)
  [PulseStep] -> Scirpt Test/6(PulseStep)
  SkipStep/1 -> Scirpt Test/15(SkipStep)
  ProfileSchedule/4(ProfileScheduleParameters) -> Scirpt Test/13(ProfileScheduleParameterIn)
  ProfileSchedule/3(ProfileScheduleType) -> Scirpt Test/12(ProfileScheduleTypeIn)
  [SOCTarget] -> Charging_Mode/4(SOCTarget)
  ProfileSchedule/1(SuiteSchedule) -> Scirpt Test/10(SuiteSchedule)
  Scirpt Test/9(ProfileScheduleType) -> ProfileScheduleBreakout/2(Type)
  Scirpt Test/12(Suite) -> Terminator6/1
  Scirpt Test/8(ProfileScheduleClass) -> ProfileScheduleBreakout/1(Class)
  Scirpt Test/10(ProfileScheduleParameter) -> ProfileScheduleBreakout/3(Parameter)
  Scirpt Test/11(Step) -> ProfileScheduleBreakout/4(Step)  "MainStep"
  ProfileScheduleBreakout/1(ActiveClass) -> Terminator1/1
  ProfileScheduleBreakout/2(ActiveType) -> Terminator3/1
  PackVolt_MaxCell/1 -> [PackVolt_MaxCell]
  Data Store Read6/1 -> Scirpt Test/16(EnblSOCTerm)
  Data Store Read5/1 -> Scirpt Test/17(SOCDeplete)
  Scirpt Test/13(ResetRun) -> [ResetRunSuite]
  PackVolt_MinCell/1 -> [PackVolt_MinCell]
  [PackVolt_MaxCell] -> Capacity Test/3(MaxCall_PackVolt)
  [PackVolt_MinCell] -> Capacity Test/4(MinCall_PackVolt)
  [Voltage] -> Capacity Test/5(CyclerVoltage)
  Capacity Test/3(CapStep) -> [CapStep]
  [CapStep] -> Scirpt Test/18(CapStep)
  [CS_SwitchMode] -> Drive_Profile/7(CSSwitch)
  Scirpt Test/14(EndStep) -> [EndStep]
  [Current] -> OCV Test/1(Current)
  [Voltage] -> OCV Test/2(Voltage)
  [Indicator] -> Compare To Constant4/1
  Compare To Constant4/1 -> Logical Operator6/1
  Logical Operator6/1 -> OCV Test/Enable
  OCV Test/2(Mode_Cntrl_OCV) -> [OCVMode]
  OCV Test/1(Profile_Data_OCV) -> [OCVData]
  Scirpt Test/6(ResetSOC) -> [ResetSOCSuite]
  Merge2/1 -> ResetSOC/1
  [ResetSOCSuite] -> Merge2/1
  OCV Test/4(ResetSOC) -> [ResetSOC]
  OCV Test/3(OCVStep) -> [OCVStep]
  [ResetSOC] -> Merge2/2
  OCV Test/5(ResetRun) -> [ResetRunOCV]
  [ResetRunSuite] -> Merge3/1
  [ResetRunOCV] -> Merge3/2
  Merge3/1 -> Data Store Write/1
  [OCVStep] -> Scirpt Test/19(OCVStep)
  Scirpt Test/1(VoltTarget) -> VoltTarget/1
  Scirpt Test/15(SOCTarget) -> Unit Delay5/1
  [PackVolt_MaxCell] -> Charging_Mode/5(PackVolt_MaxCell)
  [PackVolt_MinCell] -> Charging_Mode/6(PackVolt_MinCell)
  Unit Delay5/1 -> [SOCTarget]
  [CS_SwitchMode] -> Scirpt Test/20(SwitchMode)
  ProfileSchedule/5(ProfileScheduleParameters2) -> Scirpt Test/14(ProfileScheduleParameterIn2)
  [StartTime] -> Unit Delay9/1
  [EndTime] -> Unit Delay10/1
  Unit Delay9/1 -> Drive_Profile/8(StartTime)
  Unit Delay10/1 -> Drive_Profile/9(EndTime)
  Scirpt Test/16(StartTime) -> [StartTime]
  Scirpt Test/17(EndTime) -> [EndTime]
  [SOC] -> Scirpt Test/2(SOC)
  [SOC] -> Charging_Mode/7(SOC)
  [Indicator] -> Compare To Constant6/1
  Compare To Constant6/1 -> Logical Operator7/1
  Logical Operator7/1 -> Idle/Enable
  Idle/1(Profile_Data_idle) -> [IdleData]
  Idle/2(Mode_Cntrl_idle) -> [IdleMode]
  Idle/3(IdleStep) -> Unit Delay11/1
  Unit Delay11/1 -> [IdleStep]
  [IdleTime] -> Idle/1(TimeRequest)
  Data Store Read17/1 -> Scirpt Test/21(FA)
  [IdleStep] -> Scirpt Test/22(IdleStep)
  Data Store Read9/1 -> Scirpt Test/23(ManualIdle)
  [PowerReq] -> Idle/2(PowerReq)
  [Indicator] -> Compare To Constant9/1
  Compare To Constant9/1 -> Logical Operator8/1
  Logical Operator8/1 -> Rate/Enable
  [CurrLim] -> Rate/1(CurrLimit)
  [Rate] -> Rate/2(Rate)
  [Direction] -> Rate/3(Direction)
  Rate/1(Profile_Data_rate) -> [RateData]
  Rate/2(Mode_Cntrl_rate) -> [RateMode]
  Unit Delay13/1 -> [RateStep]
  Scirpt Test/21(Rate) -> [Rate]
  Scirpt Test/22(CurrLim) -> [CurrLim]
  [RateStep] -> Scirpt Test/24(RateStep)
  Rate/3(RateStep) -> Unit Delay13/1
  Scirpt Test/18(IdleTime) -> [IdleTime]
  Scirpt Test/19(PowerReq) -> [PowerReq]
  Scirpt Test/7(SuiteStep) -> Terminator4/1
  Logical Operator9/1 -> Increment/Enable
  [Indicator] -> Compare To Constant7/1
  Compare To Constant7/1 -> Logical Operator9/1
  [Voltage] -> Increment/1(Voltage)
  [PackVolt_MinCell] -> Increment/2(PackVolt_MinCell)
  Increment/3(IncrementStep) -> Unit Delay14/1
  Unit Delay14/1 -> [IncrementStep]
  [IncrementStep] -> Scirpt Test/25(IncrementStep)
  Scirpt Test/3(IndicatorSF) -> IndicatorSF/1  "IndicatorSF"
  [ChargingMode] -> Merge1/1
  [DriveMode] -> Merge1/2
  [StandbyMode] -> Merge1/3
  [CapacityMode] -> Merge1/4
  [HPPCMode] -> Merge1/5
  [PulseMode] -> Merge1/6
  [OCVMode] -> Merge1/7
  [IdleMode] -> Merge1/8
  [RateMode] -> Merge1/9
  [ChargingData] -> Merge4/1
  [DriveData] -> Merge4/2
  [CapData] -> Merge4/3
  [HPPCData] -> Merge4/4
  [PulseData] -> Merge4/5
  [OCVData] -> Merge4/6
  [IdleData] -> Merge4/7
  [RateData] -> Merge4/8
  [IncrementData] -> Merge4/9
  Increment/1(Profile_Data_inc) -> [IncrementData]
  Increment/2(Mode_Cntrl_inc) -> [IncrementMode]
  [IncrementMode] -> Merge1/10
  Indicator/1 -> [Indicator]
  Data Store Read7/1 -> Logical Operator2/2
  Data Store Read8/1 -> Logical Operator3/2
  Data Store Read11/1 -> Logical Operator4/2
  Data Store Read12/1 -> Logical Operator5/2
  Data Store Read13/1 -> Logical Operator6/2
  Data Store Read14/1 -> Logical Operator7/2
  Data Store Read15/1 -> Logical Operator8/2
  Data Store Read16/1 -> Logical Operator9/2
  CS_ModeSwitch/1 -> [CS_SwitchMode]
  Data Store Read1/1 -> Logical Operator11/1
  Compare To Constant2/1 -> Logical Operator10/1
  Logical Operator11/1 -> Logical Operator10/2
  Logical Operator10/1 -> Standby_Sub/Enable
  Merge1/1 -> Profile_Mode/1  "Mode"
  [ESTOP] -> Logical Operator10/3
  ESTOP/1 -> [ESTOP]
  SOC/1 -> [SOC]
  Voltage_Cntrl/1 -> [Voltage_Cntrl]
  Current_Cntrl/1 -> [Current_Cntrl]
  [Voltage_Cntrl] -> Charging_Mode/8(Voltage_Cntrl)
  [Current_Cntrl] -> Charging_Mode/9(Current_Cntrl)
  Scirpt Test/23(SetChamberT_ToBatTemp) -> SetChamberT_ToBatTemp/1  "SetChamberT_ToBatTemp"
  Scirpt Test/20(CurrentReq) -> [CurrentReq]
  [CurrentReq] -> Idle/3(CurrentReq)
  Scirpt Test/24(Idle_Type) -> [Idle_Type]
  [Idle_Type] -> Idle/4(Idle_Type)
  Capacity Test/4(ResetSOCFlg) -> [ResetSOCFlg]
  [ResetSOCFlg] -> Merge2/3

== system HIL_Testing_SW_amantest/LionsHeart/FeaturePresentation/Safety/Subsystem ==
  ContactorLine : Inport  OutDataType=fixdt(1, 16)  OutScaling=2^0
  ContactorStatus : Inport  Port=2  OutDataType=fixdt(1, 16)  OutScaling=2^0
  Chargemode : Inport  Port=3  OutDataType=fixdt(1, 16)  OutScaling=2^0
  Compare To Constant7 : simulink/Logic and Bit Operations/Compare To Constant  SystemSampleTime=-1  relop===  const=0  LogicOutDataTypeMode=uint8  ZeroCross=off
  Data Store Read : DataStoreRead  DataStoreName=ContactorOverride  SampleTime=0
  Default : Constant  Value=0  OutDataType=fixdt(1, 16)  OutScaling=2^0
  Default1 : Constant  Value=0  OutDataType=fixdt(1, 16)  OutScaling=2^0  OutDataTypeStr=Inherit: Inherit via back propagation
  Logical Operator : Logic  AllPortsSameDT=off  OutDataTypeMode=boolean  OutDataTypeStr=boolean
  SafetyCont : Switch  Threshold=0.5  OutDataType=fixdt(1, 16)  OutScaling=2^0
  Switch : Switch  OutDataType=fixdt(1, 16)  OutScaling=2^0
  CntLine : Outport  OutDataType=fixdt(1, 16)  OutScaling=2^0
  CntStat : Outport  Port=2  OutDataType=fixdt(1, 16)  OutScaling=2^0
  wires:
  ContactorStatus/1 -> Compare To Constant7/1
  Chargemode/1 -> SafetyCont/2
  Default/1 -> SafetyCont/1
  SafetyCont/1 -> Logical Operator/2
  Compare To Constant7/1 -> Logical Operator/1
  ContactorLine/1 -> SafetyCont/3, CntLine/1
  Logical Operator/1 -> Switch/3
  Switch/1 -> CntStat/1
  Data Store Read/1 -> Switch/2
  Default1/1 -> Switch/1

== system HIL_Testing_SW_amantest/LionsHeart/Input Processing/Current Processing/ChargeTerminationCurrent ==
  BatteryTemp : Inport  OutDataType=fixdt(1, 16)  OutScaling=2^0
  CurrentTermination : Lookup  InputValues=KnBSER_T_BlendTempAxis  Table=KtBSER_I_IchgThrsh  OutDataType=fixdt(1, 16)  OutScaling=2^0
  Data Store Read : DataStoreRead  DataStoreName=ManualCurrentTerm  SampleTime=0
  Data Store Read1 : DataStoreRead  DataStoreName=ManualCurrentTerm_Switch  SampleTime=0
  Data Store Write25 : DataStoreWrite  DataStoreName=TerminationCurrent  SampleTime=-1
  Switch2 : Switch  Criteria=u2 > Threshold  OutDataType=fixdt(1, 16)  OutScaling=2^0  OutDataTypeStr=Inherit: Inherit via back propagation
  wires:
  BatteryTemp/1 -> CurrentTermination/1
  CurrentTermination/1 -> Switch2/3
  Data Store Read/1 -> Switch2/1
  Switch2/1 -> Data Store Write25/1
  Data Store Read1/1 -> Switch2/2

== system HIL_Testing_SW_amantest/LionsHeart/Input Processing/Current Processing/Current Control Select ==
  PackCurrent : Inport  OutDataType=fixdt(1, 16)  OutScaling=2^0
  CyclerCurrent : Inport  Port=2  OutDataType=fixdt(1, 16)  OutScaling=2^0
  SOCTerm1 : DataStoreRead  DataStoreName=UsePackSensor  SampleTime=0
  Switch5 : Switch  Criteria=u2 > Threshold  Threshold=0.5  OutDataType=fixdt(1, 16)  OutScaling=2^0  OutDataTypeStr=Inherit: Inherit via back propagation
  Current_Cntrl : Outport  OutDataType=fixdt(1, 16)  OutScaling=2^0
  wires:
  CyclerCurrent/1 -> Switch5/3
  PackCurrent/1 -> Switch5/1
  Switch5/1 -> Current_Cntrl/1
  SOCTerm1/1 -> Switch5/2

== system HIL_Testing_SW_amantest/LionsHeart/Input Processing/Current Processing/CurrentLimit_Charge ==
  BatteryTemp : Inport  OutDataType=fixdt(1, 16)  OutScaling=2^0
  HVBatCrntUpLmt_CAN : Inport  Port=2  OutDataType=fixdt(1, 16)  OutScaling=2^0
  ChrgCurrLim : Lookup  InputValues=[-30 -20 -10 0 10 20 30 40 50]  Table=[ChrgCurrLim]  OutDataType=fixdt(1, 16)  OutScaling=2^0
  Data Store Read : DataStoreRead  DataStoreName=CLim_Switch  SampleTime=0
  Data Store Write15 : DataStoreWrite  DataStoreName=ChrgCurrLim  SampleTime=-1
  Switch1 : Switch  Threshold=.5  OutDataType=fixdt(1, 16)  OutScaling=2^0  OutDataTypeStr=Inherit: Inherit via back propagation
  wires:
  BatteryTemp/1 -> ChrgCurrLim/1
  Data Store Read/1 -> Switch1/2
  ChrgCurrLim/1 -> Switch1/1
  HVBatCrntUpLmt_CAN/1 -> Switch1/3
  Switch1/1 -> Data Store Write15/1

== system HIL_Testing_SW_amantest/LionsHeart/Input Processing/Current Processing/CurrentLimit_Discharge ==
  BatteryTemp : Inport  OutDataType=fixdt(1, 16)  OutScaling=2^0
  HVBatCrntLwLmt_CAN : Inport  Port=2  OutDataType=fixdt(1, 16)  OutScaling=2^0
  Data Store Read : DataStoreRead  DataStoreName=CLim_Switch  SampleTime=0
  Data Store Write16 : DataStoreWrite  DataStoreName=DschrgCurrLim  SampleTime=-1
  DschrgCurrLim : Lookup  InputValues=[-30 -20 -10 0 10 20 30 40 50]  Table=[DschrgCurrLim]  OutDataType=fixdt(1, 16)  OutScaling=2^0
  Switch1 : Switch  Threshold=.5  OutDataType=fixdt(1, 16)  OutScaling=2^0  OutDataTypeStr=Inherit: Inherit via back propagation
  wires:
  BatteryTemp/1 -> DschrgCurrLim/1
  Data Store Read/1 -> Switch1/2
  DschrgCurrLim/1 -> Switch1/1
  Switch1/1 -> Data Store Write16/1
  HVBatCrntLwLmt_CAN/1 -> Switch1/3
